simulink subsystem "RAM"  (R2024b)
settings: Solver=VariableStepAuto  StartTime=0.0  StopTime=10.0  RelTol=1e-3
values from neighbouring files (symbols this model uses):
  modelStopCondition = "tohost"    [initSimuRISC.m]
  tohost_address = hex2dec('1000')    [initSimuRISC.m]
libraries: hdlsllib x2, simulink x2
settings Model: Creator=stefano  LastModifiedBy=stefano

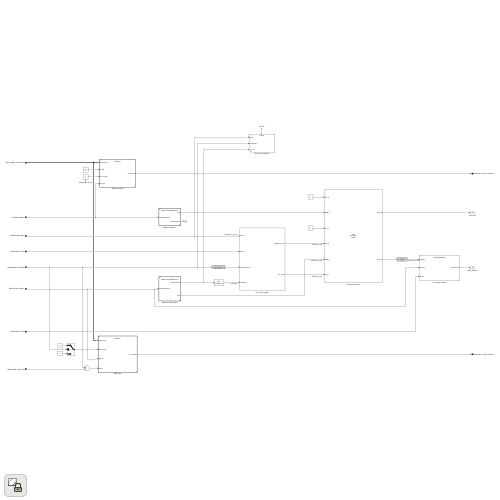
[thumbnail: Simulink's stored preview of the top-level diagram]
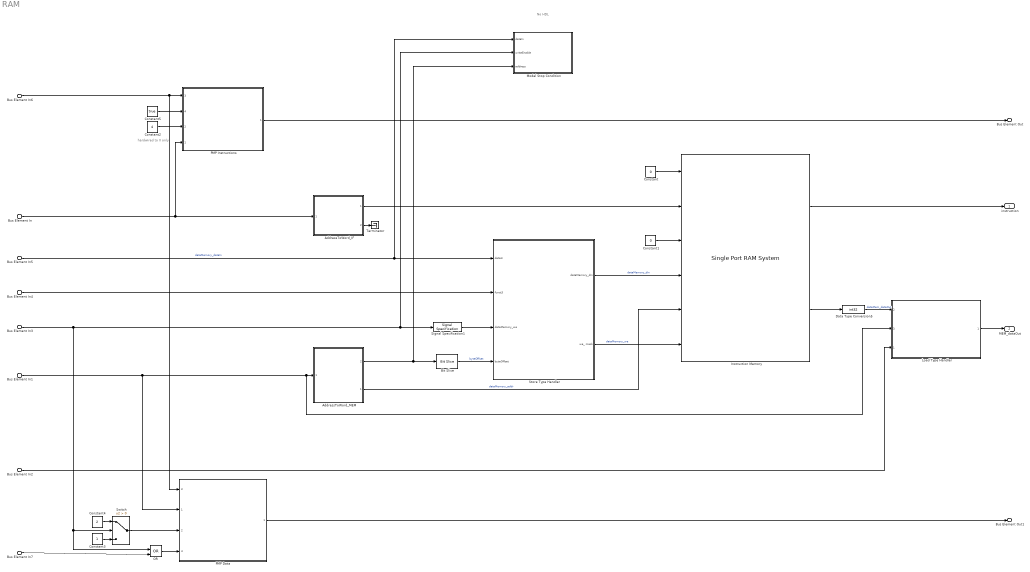
== system RAM ==
  note: hardwired to X only
  note: No HDL
  Bus Element In6 : Inport  PortName=BUS_dataRtn  Element=PMPConfig
  Bus Element In : Inport  Port=2  PortName=IFToRAM  Element=address
  Bus Element In1 : Inport  Port=3  PortName=MEMToRAM  Element=address
  Bus Element In2 : Inport  Port=3  PortName=MEMToRAM  Element=funct3
  Bus Element In4 : Inport  Port=3  PortName=MEMToRAM  Element=funct3
  Bus Element In3 : Inport  Port=3  PortName=MEMToRAM  Element=memWrite
  Bus Element In5 : Inport  Port=3  PortName=MEMToRAM  Element=dataIn
  Bus Element In7 : Inport  Port=3  PortName=MEMToRAM  Element=memRead
  AddressToWord_IF : Subsystem  TreatAsAtomicUnit=on  ReferencedSubsystem=AddressToWordSelector
  AddressToWord_MEM : Subsystem  TreatAsAtomicUnit=on  ReferencedSubsystem=AddressToWordSelector
      settings: PortSchema="{\"entries\":[{\"content\":{\"sides\":[{\"content\":{\"connectorIds\":[\"In1\"]},\"type\":\"ConnectorPlacement.EquallySpacedRectSide\",\"uuid\":\"bdfc407e-e30c-446a-8a17-95e99ed9324e\"},{\"content\":{\"connectorIds\":[\"Out2\",\"Out1\"],\"side\":\"RIGHT\"},\"type\":\"ConnectorPlacement.EquallySpacedRectSide\",\"uuid\":\"e65c5857-7630-49d4-b3b9-4bfd850ce567\"},{\"content\":{\"side\":\"TOP\"},\"type\":\"ConnectorPlacement.EquallySpacedRectSide\",\"uuid\":\"02f27867-aa47-4e09-b1e6-ae0b6a65408b\"}]},\"type\":\"ConnectorPlacement.EquallySpacedConnector\",\"uuid\":\"fdffddc1-4054-4108-82ac-b2549a0fa510\"}],\"packageUris\":[\"http://schema.mathworks.com/mf0/Connector/R2020b\"],\"version\":\"1.0\"}"
  Bit Slice : hdlsllib/Logic and Bit Operations/Bit Slice  lidx=1  ridx=0
  Constant : Constant  Value=0  OutDataTypeStr=uint32  SampleTime=-1
  Constant1 : Constant  Value=0  OutDataTypeStr=fixdt(0,4,0)  SampleTime=-1
  Constant2 : Constant  Value=4  OutDataTypeStr=fixdt(0,3,0)  SampleTime=-1
  Constant3 : Constant  Value=1  OutDataTypeStr=fixdt(0,3,0)  SampleTime=-1
  Constant4 : Constant  Value=2  OutDataTypeStr=fixdt(0,3,0)  SampleTime=-1
  Constant5 : Constant  Value=true  OutDataTypeStr=boolean  SampleTime=-1
  Data Type Conversion5 : DataTypeConversion  OutDataTypeStr=int32  SaturateOnIntegerOverflow=off  RndMeth=Floor
  Instruction Memory : hdlsllib/HDL RAMs/Single Port RAM System  RAMType=True dual port  AsyncRead=off  WriteOutputValue=Old data  RAMInitialValue=memoryData  allowBusInputs=off  WritesHaveOutput=on  NumReads=0  NumWrites=1  SimulateUsing=Code generation  ModelRAMDelay=on
  Load Type Handler : Subsystem  ReferencedSubsystem=LoadTypeHandler
      settings: PortSchema="{\"entries\":[{\"content\":{\"sides\":[{\"content\":{\"connectorIds\":[\"In2\",\"In3\",\"In1\"]},\"type\":\"ConnectorPlacement.EquallySpacedRectSide\",\"uuid\":\"476fc81f-d679-4801-b269-a822056a7620\"},{\"content\":{\"connectorIds\":[\"Out1\"],\"side\":\"RIGHT\"},\"type\":\"ConnectorPlacement.EquallySpacedRectSide\",\"uuid\":\"e81ff414-cf8b-4e84-b170-6f68c2bd00ae\"},{\"content\":{\"side\":\"TOP\"},\"type\":\"ConnectorPlacement.EquallySpacedRectSide\",\"uuid\":\"7cf0cb5e-f5c9-4ba1-9748-8e063d9d1305\"}]},\"type\":\"ConnectorPlacement.EquallySpacedConnector\",\"uuid\":\"b2bc2daa-80da-419a-b4be-1931c672cf78\"}],\"packageUris\":[\"http://schema.mathworks.com/mf0/Connector/R2020b\"],\"version\":\"1.0\"}"
  Model Stop Condition : Subsystem  Variant=on  VariantControl=Subsystem  AllowZeroVariantControls=on
  OR : Logic  Operator=OR  IconShape=distinctive  AllPortsSameDT=off  OutDataTypeStr=boolean
  PMP Data : Subsystem  TreatAsAtomicUnit=on  ReferencedSubsystem=PMPUnit
      settings: PortSchema="{\"entries\":[{\"content\":{\"sides\":[{\"content\":{\"connectorIds\":[\"In3\",\"In1\",\"In2\",\"In4\"]},\"type\":\"ConnectorPlacement.EquallySpacedRectSide\",\"uuid\":\"16ef9972-eb69-48d0-b551-1ee41a9e1bb7\"},{\"content\":{\"connectorIds\":[\"Out1\"],\"side\":\"RIGHT\"},\"type\":\"ConnectorPlacement.EquallySpacedRectSide\",\"uuid\":\"f7c5c781-8055-443d-9c43-a55f5962ee47\"},{\"content\":{\"side\":\"TOP\"},\"type\":\"ConnectorPlacement.EquallySpacedRectSide\",\"uuid\":\"259daa94-3e35-4c17-a598-89751261d251\"}]},\"type\":\"ConnectorPlacement.EquallySpacedConnector\",\"uuid\":\"7aaedc52-0cc8-4991-85e0-8ffd081d954f\"}],\"packageUris\":[\"http://schema.mathworks.com/mf0/Connector/R2020b\"],\"version\":\"1.0\"}"
  PMP Instructions : Subsystem  TreatAsAtomicUnit=on  ReferencedSubsystem=PMPUnit
      settings: PortSchema="{\"entries\":[{\"content\":{\"sides\":[{\"content\":{\"connectorIds\":[\"In3\",\"In4\",\"In2\",\"In1\"]},\"type\":\"ConnectorPlacement.EquallySpacedRectSide\",\"uuid\":\"16ef9972-eb69-48d0-b551-1ee41a9e1bb7\"},{\"content\":{\"connectorIds\":[\"Out1\"],\"side\":\"RIGHT\"},\"type\":\"ConnectorPlacement.EquallySpacedRectSide\",\"uuid\":\"f7c5c781-8055-443d-9c43-a55f5962ee47\"},{\"content\":{\"side\":\"TOP\"},\"type\":\"ConnectorPlacement.EquallySpacedRectSide\",\"uuid\":\"259daa94-3e35-4c17-a598-89751261d251\"}]},\"type\":\"ConnectorPlacement.EquallySpacedConnector\",\"uuid\":\"7aaedc52-0cc8-4991-85e0-8ffd081d954f\"}],\"packageUris\":[\"http://schema.mathworks.com/mf0/Connector/R2020b\"],\"version\":\"1.0\"}"
  Signal Specification1 : SignalSpecification  OutDataTypeStr=boolean
  Store Type Handler : Subsystem
  Switch : Switch  Criteria=u2 > Threshold  SaturateOnIntegerOverflow=off  InputSameDT=off
  Terminator : Terminator
  instruction : Outport
  MEM_dataOut : Outport  Port=2
  Bus Element Out : Outport  Port=3  PortName=PMPFaults  Element=instrAccessFault
  Bus Element Out1 : Outport  Port=3  PortName=PMPFaults  Element=loadAccessFault
  wires:
  Constant/1 -> Instruction Memory/1
  Constant1/1 -> Instruction Memory/3
  Instruction Memory/1 -> instruction/1
  Store Type Handler/2(we_ mask) -> Instruction Memory/6  "dataMemory_we"
  Data Type Conversion5/1 -> Load Type Handler/2  "dataMem_dataOut"
  Load Type Handler/1 -> MEM_dataOut/1
  Store Type Handler/1(dataMemory_din) -> Instruction Memory/4  "dataMemory_din"
  Instruction Memory/2 -> Data Type Conversion5/1
  Bus Element In2/1 -> Load Type Handler/1
  Bus Element In5/1 -> Model Stop Condition/1(dataIn), Store Type Handler/1(dataIn)  "dataMemory_dataIn"
  Signal Specification1/1 -> Store Type Handler/3(dataMemory_we)
  Bus Element In4/1 -> Store Type Handler/2(funct3)
  Bus Element In3/1 -> Signal Specification1/1, Model Stop Condition/2(writeEnable), Switch/2, OR/1
  Bit Slice/1 -> Store Type Handler/4(byteOffset)  "byteOffset"
  Bus Element In1/1 -> PMP Data/1, AddressToWord_MEM/1, Load Type Handler/3
  Bus Element In/1 -> PMP Instructions/1, AddressToWord_IF/1
  AddressToWord_IF/1 -> Instruction Memory/2
  AddressToWord_IF/2 -> Terminator/1
  AddressToWord_MEM/2 -> Bit Slice/1, Model Stop Condition/3(address)
  AddressToWord_MEM/1 -> Instruction Memory/5  "dataMemory_addr"
  Bus Element In6/1 -> PMP Instructions/3, PMP Data/3
  Constant2/1 -> PMP Instructions/2
  PMP Instructions/1 -> Bus Element Out/1
  Constant3/1 -> Switch/3
  Constant4/1 -> Switch/1
  PMP Data/1 -> Bus Element Out1/1
  OR/1 -> PMP Data/4
  Bus Element In7/1 -> OR/2
  Switch/1 -> PMP Data/2
  Constant5/1 -> PMP Instructions/4

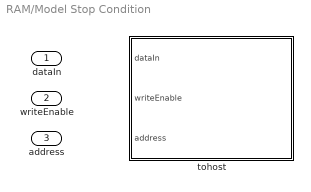
== system RAM/Model Stop Condition ==
  dataIn : Inport
  writeEnable : Inport  Port=2
  address : Inport  Port=3
  tohost : Subsystem  VariantControl="strcmp(modelStopCondition, \"tohost\")"

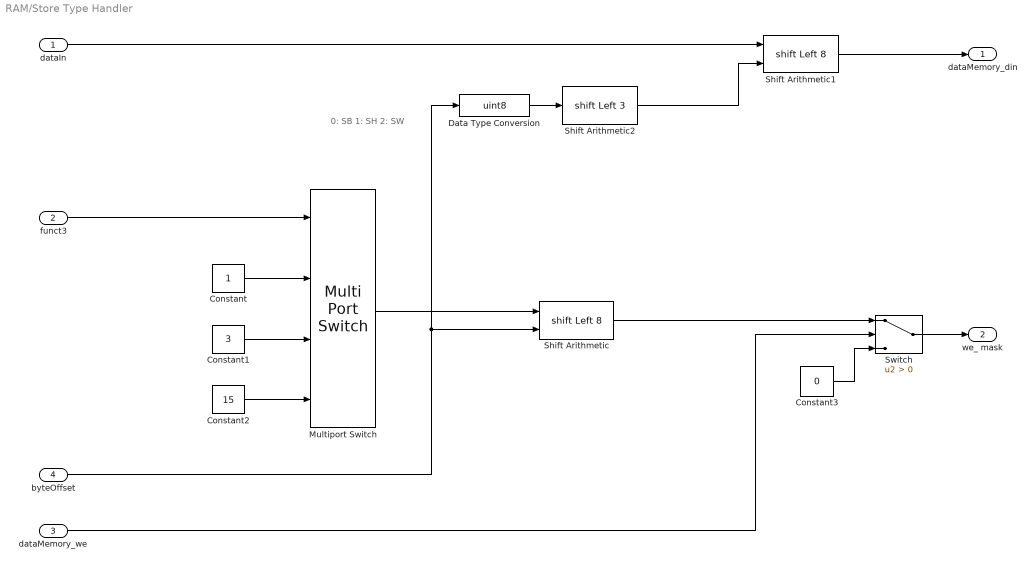
== system RAM/Store Type Handler ==
  note: 0: SB
      | 1: SH
      | 2: SW
  dataIn : Inport
  funct3 : Inport  Port=2
  dataMemory_we : Inport  Port=3
  byteOffset : Inport  Port=4
  Constant : Constant  OutDataTypeStr=fixdt(0,4,0)  SampleTime=-1
  Constant1 : Constant  Value=3  OutDataTypeStr=fixdt(0,4,0)  SampleTime=-1
  Constant2 : Constant  Value=15  OutDataTypeStr=fixdt(0,4,0)  SampleTime=-1
  Constant3 : Constant  Value=0  OutDataTypeStr=fixdt(0,4,0)  SampleTime=-1
  Data Type Conversion : DataTypeConversion  OutDataTypeStr=uint8  SaturateOnIntegerOverflow=off  RndMeth=Floor
  Multiport Switch : MultiPortSwitch  DataPortOrder=Zero-based contiguous  DataPortIndices={0,1,2,4,5}  DiagnosticForDefault=None  zeroidx=on  SaturateOnIntegerOverflow=off  InputSameDT=off
  Shift Arithmetic : ArithShift  BitShiftNumberSource=Input port  BitShiftNumber=8  BitShiftDirection=Left
      settings: InputPortMap=u0,p1
  Shift Arithmetic1 : ArithShift  BitShiftNumberSource=Input port  BitShiftNumber=8  BitShiftDirection=Left
      settings: InputPortMap=u0,p1
  Shift Arithmetic2 : ArithShift  BitShiftNumber=3  BitShiftDirection=Left
  Switch : Switch  Criteria=u2 > Threshold  SaturateOnIntegerOverflow=off  InputSameDT=off
  dataMemory_din : Outport
  we_ mask : Outport  Port=2
  wires:
  Multiport Switch/1 -> Shift Arithmetic/1
  Constant1/1 -> Multiport Switch/3
  Constant/1 -> Multiport Switch/2
  funct3/1 -> Multiport Switch/1
  Shift Arithmetic/1 -> Switch/1
  byteOffset/1 -> Shift Arithmetic/2, Data Type Conversion/1
  dataMemory_we/1 -> Switch/2
  Switch/1 -> we_ mask/1
  Constant2/1 -> Multiport Switch/4
  Constant3/1 -> Switch/3
  dataIn/1 -> Shift Arithmetic1/1
  Shift Arithmetic1/1 -> dataMemory_din/1
  Data Type Conversion/1 -> Shift Arithmetic2/1
  Shift Arithmetic2/1 -> Shift Arithmetic1/2

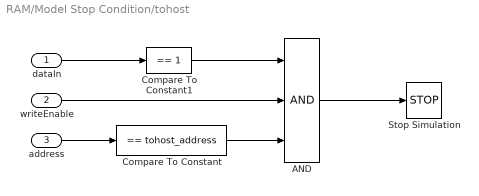
== system RAM/Model Stop Condition/tohost ==
  dataIn : Inport
  writeEnable : Inport  Port=2
  address : Inport  Port=3
  AND : Logic  Inputs=3  IconShape=distinctive  AllPortsSameDT=off  OutDataTypeStr=boolean
  Compare To Constant : simulink/Logic and Bit Operations/Compare To Constant  relop===  const=tohost_address  OutDataTypeStr=boolean
  Compare To Constant1 : simulink/Logic and Bit Operations/Compare To Constant  relop===  const=1  OutDataTypeStr=boolean
  Stop Simulation : Stop
  wires:
  writeEnable/1 -> AND/2
  dataIn/1 -> Compare To Constant1/1
  AND/1 -> Stop Simulation/1
  address/1 -> Compare To Constant/1
  Compare To Constant1/1 -> AND/1
  Compare To Constant/1 -> AND/3
